simulink model "EC_core_control"  (R2023b)
settings: configuration reference "ctrl_tsk_conf" (kept outside this file)
undefined symbols (not defined in the file): DC_ff_max, DC_ff_min, Max_DC_limit, Tr_max_v, Trx_Ratio
libraries: eeGeneralControl x3, simulink x1
settings Model: DataDictionary=fmuGenerationDictionay.sldd  ModifiedByFormat=Third Equation Ltd  Creator=Third Equation Ltd  LastModifiedBy=Third Equation Ltd
settings ConfigSetRef: SourceName=ctrl_tsk_conf

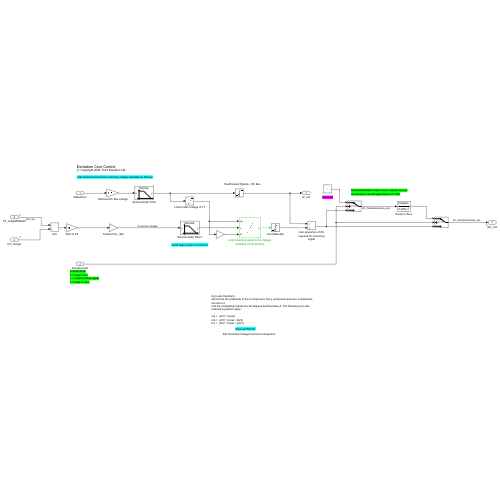
[thumbnail: Simulink's stored preview of the top-level diagram]
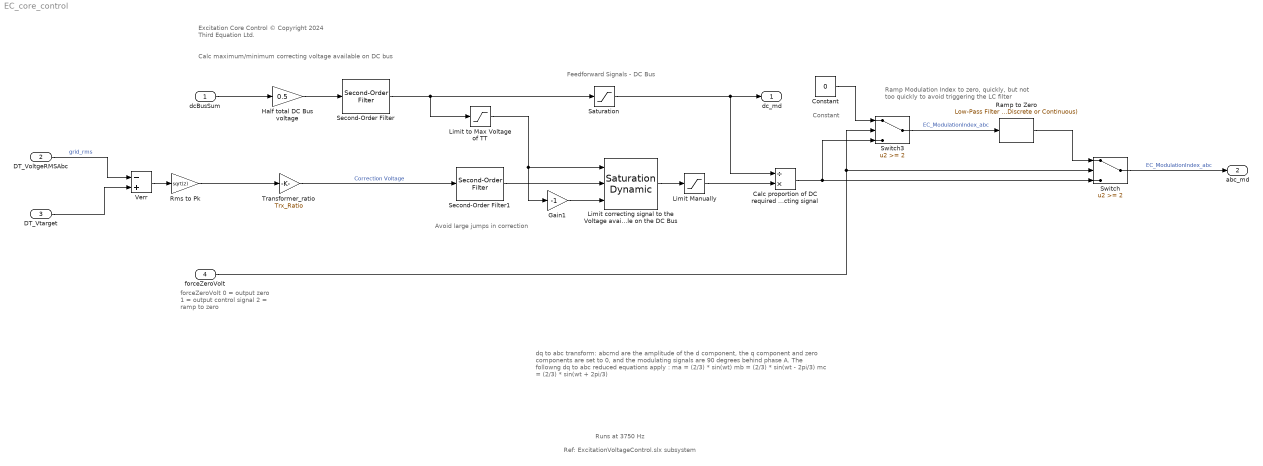
== system EC_core_control ==
  note: Feedforward Signals - DC Bus
  note: Calc maximum/minimum correcting voltage available on DC bus
  note: Avoid large jumps in correction
  note: Runs at 3750 Hz
  note: Excitation Core Control
      | © Copyright 2024 Third Equation Ltd.
  note: Ref: ExcitationVoltageControl.slx subsystem
  note: dq to abc transform:
      | abcmd are the amplitude of the d component, the q component and zero components
      | are set to 0,
      | and the modulating signals are 90 degrees behind phase A. The followng dq to abc reduced equations apply :
      |
      | ma =  (2/3) * sin(wt)
      | mb =  (2/3) * sin(wt - 2pi/3)
      | mc =  (2/3) * sin(wt + 2pi/3)
  note: forceZeroVolt
      | 0 = output zero
      | 1 = output control signal
      | 2 = ramp to zero
  note: Constant
  note: Ramp Modulation Index to zero, quickly, but not
      | too quickly to avoid triggering the LC filter
  dcBusSum : Inport  OutDataTypeStr=single  Unit=V  PortDimensions=1
  DT_VoltgeRMSAbc : Inport  Port=2  OutDataTypeStr=single  Unit=V  PortDimensions=3
  DT_Vtarget : Inport  Port=3  OutDataTypeStr=single  Unit=V  PortDimensions=3
  forceZeroVolt : Inport  Port=4  OutDataTypeStr=uint8  PortDimensions=1
  Calc proportion of DC required for correcting signal : Product  Inputs=/*  OutDataTypeStr=single
  Constant : Constant  Value=0  OutDataTypeStr=single
  Gain1 : Gain  Gain=-1  ParamDataTypeStr=single  OutDataTypeStr=single
  Half total DC Bus voltage : Gain  Gain=0.5  ParamDataTypeStr=single  OutDataTypeStr=single
  Limit Manually : Saturate  UpperLimit=Max_DC_limit  LowerLimit=-Max_DC_limit  OutDataTypeStr=single
  Limit correcting signal to the Voltage available on the DC Bus : simulink/Discontinuities/Saturation Dynamic  OutMin=[]  OutMax=[]  OutDataTypeStr=single  OutputDataTypeScalingMode=single  OutDataType=fixdt(1, 16)  OutScaling=2^-10  DoSatur=off
  Limit to Max Voltage of TT : Saturate  UpperLimit=Tr_max_v  LowerLimit=0  OutDataTypeStr=single
  Ramp to Zero : eeGeneralControl/Low-Pass Filter (Discrete or Continuous)  K=1  T=0.005  B=inf  A=-inf  init_option=Inherited from block input  x0=0  Ts=-1
  Rms to Pk : Gain  Gain=sqrt(2)  ParamDataTypeStr=single  OutDataTypeStr=single
  Saturation : Saturate  UpperLimit=DC_ff_max  LowerLimit=DC_ff_min  OutDataTypeStr=single
  Second-Order Filter : eeGeneralControl/Second-Order Filter  FilterType=Low-pass  fn=single(1)  Zeta=single(0.707)  Ts=-1  A0=0  Ph0=0  f0=0  b0=0
  Second-Order Filter1 : eeGeneralControl/Second-Order Filter  FilterType=Low-pass  fn=single(1)  Zeta=single(0.707)  Ts=-1  A0=0  Ph0=0  f0=0  b0=0
  Switch : Switch  Threshold=2  OutDataTypeStr=single  SaturateOnIntegerOverflow=off  InputSameDT=off
  Switch3 : Switch  Threshold=2  OutDataTypeStr=single  SaturateOnIntegerOverflow=off  InputSameDT=off
  Transformer_ratio : Gain  Gain=Trx_Ratio
  Verr : Sum  Inputs=-+  OutDataTypeStr=single  AccumDataTypeStr=single
  dc_md : Outport  OutDataTypeStr=single  Unit=1  PortDimensions=1
  abc_md : Outport  Port=2  OutDataTypeStr=single  Unit=1  PortDimensions=3
  wires:
  Saturation/1 -> Calc proportion of DC required for correcting signal/1, dc_md/1
  Gain1/1 -> Limit correcting signal to the Voltage available on the DC Bus/3
  dcBusSum/1 -> Half total DC Bus voltage/1
  Limit to Max Voltage of TT/1 -> Gain1/1, Limit correcting signal to the Voltage available on the DC Bus/1
  Second-Order Filter1/1 -> Limit correcting signal to the Voltage available on the DC Bus/2
  Second-Order Filter/1 -> Limit to Max Voltage of TT/1, Saturation/1
  Limit Manually/1 -> Calc proportion of DC required for correcting signal/2
  Half total DC Bus voltage/1 -> Second-Order Filter/1
  Transformer_ratio/1 -> Second-Order Filter1/1  "Correction Voltage"
  Limit correcting signal to the Voltage available on the DC Bus/1 -> Limit Manually/1
  forceZeroVolt/1 -> Switch/2, Switch3/2
  Switch/1 -> abc_md/1  "EC_ModulationIndex_abc"
  Switch3/1 -> Ramp to Zero/1  "EC_ModulationIndex_abc"
  Constant/1 -> Switch3/1
  Ramp to Zero/1 -> Switch/1
  Calc proportion of DC required for correcting signal/1 -> Switch/3, Switch3/3
  Rms to Pk/1 -> Transformer_ratio/1
  DT_Vtarget/1 -> Verr/2
  Verr/1 -> Rms to Pk/1
  DT_VoltgeRMSAbc/1 -> Verr/1  "grid_rms"
